simulink model "M"  (R2022b)
settings: Solver=FixedStepAuto  StartTime=0.0  StopTime=10.0  RelTol=1e-3
settings Model: Creator=86134  LastModifiedBy=86134

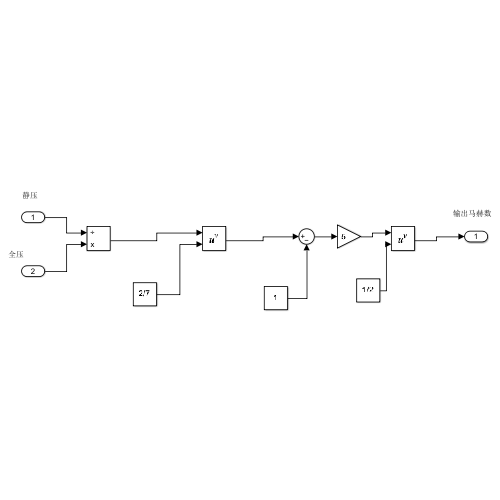
[thumbnail: Simulink's stored preview of the top-level diagram]
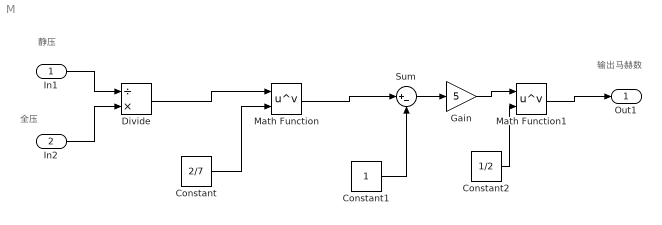
== system M ==
  note: 输出马赫数
  note: 静压
  note: 全压
  In1 : Inport
  In2 : Inport  Port=2
  Constant : Constant  Value=2/7
  Constant1 : Constant
  Constant2 : Constant  Value=1/2
  Divide : Product  Inputs=/*
  Gain : Gain  Gain=5
  Math Function : Math  Operator=pow
  Math Function1 : Math  Operator=pow
  Sum : Sum  Inputs=|+-
  Out1 : Outport
  wires:
  In2/1 -> Divide/2
  In1/1 -> Divide/1
  Divide/1 -> Math Function/1
  Constant/1 -> Math Function/2
  Constant1/1 -> Sum/2
  Math Function/1 -> Sum/1
  Sum/1 -> Gain/1
  Constant2/1 -> Math Function1/2
  Gain/1 -> Math Function1/1
  Math Function1/1 -> Out1/1
